simulink model "estimarParametros"  (R2021a)
settings: Solver=VariableStepAuto  StartTime=0.0  StopTime=10.0  RelTol=1e-3
values from neighbouring files (symbols this model uses):
  Bl0 = 0.0647    [modeloMatematico.m]    (also in motor copy.m = 0.147; motor.m = 0.05)
  Bm0 = 5.873e-9    (= 5.873e-09)    [modeloMatematico.m]    (also in motor copy.m = 5.862e-09; motor.m = 0.2)
  CL = double(subs(C_par))    [modeloMatematico.m]    (also in motor copy.m = [0 0 1/n0]; motor.m = [0 0 1/n0]; untitled.m = double(subs(C,{x1,x2,x3,u,M,g,R,L},{x10n,x20n,x30n,u0n,Mo,go)
  d0 = 0.065    [modeloMatematico.m]    (also in motor copy.m = 0.06587; motor.m = 0.1)
  g0 = 9.81    [modeloMatematico.m]    (also in motor copy.m; motor.m)
  Jl0 = 0.00000220756    (= 2.20756e-06)    [modeloMatematico.m]    (also in motor copy.m = 0.154364; motor.m = 0.02)
  Jm0 = 7.83568e-12    [modeloMatematico.m]    (also in motor copy.m = 7.83067e-12; motor.m = 0.01)
  Ki0 = 0.005119    [modeloMatematico.m]    (also in motor copy.m = 0.005012; motor.m = 2.3)
  Kv0 = 0.005119    [modeloMatematico.m]    (also in motor copy.m = 3.212e-11; motor.m = 1.5)
  L0 = 0.0013    [modeloMatematico.m]    (also in motor copy.m = 0.00051; motor.m = 0.04)
  m0 = 0.17244    [modeloMatematico.m]    (also in motor copy.m = 0.1045; motor.m = 0.1)
  n0 = 120    [modeloMatematico.m]    (also in motor copy.m; motor.m)
  R0 = 3.4    [modeloMatematico.m]    (also in motor copy.m = 3.9654; motor.m = 10)
  Vin0 = R0*x10    [modeloMatematico.m]    (also in motor copy.m; motor.m = R*x10)
  x10 = (m0*g0*d0*sin(x30))/Ki0    [modeloMatematico.m]    (also in motor copy.m = (m0*g0*d0*sin(x30/n0))/Ki0; motor.m = (m*g*d*sin(x30/n0))/Ki0)
  x20 = 0    [modeloMatematico.m]    (also in motor copy.m; motor.m; untitled.m)
  x30 = thetaL0    (= 0)    [modeloMatematico.m]    (also in motor copy.m; motor.m; untitled.m = sqrt(M*g*x10))
settings Model: OrderedModelArguments=off  Creator=hubertdelgado  LastModifiedBy=hubertdelgado

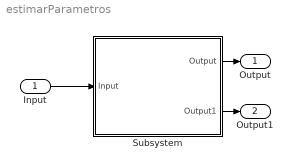
== system estimarParametros ==
  Input : Inport
  Subsystem : Subsystem
  Output : Outport
  Output1 : Outport  Port=2
  wires:
  Input/1 -> Subsystem/1(Input)
  Subsystem/1(Output) -> Output/1
  Subsystem/2(Output1) -> Output1/1

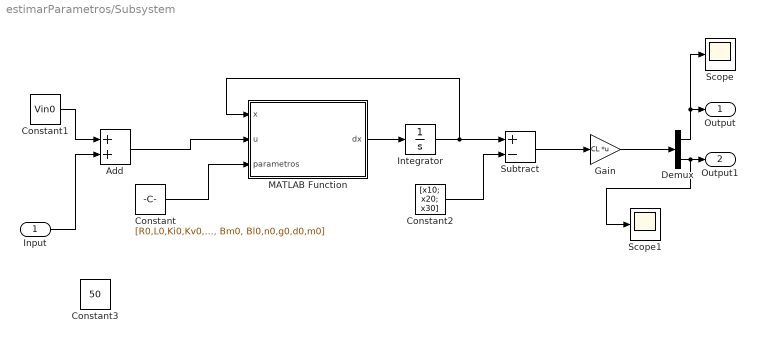
== system estimarParametros/Subsystem ==
  Input : Inport
  Add : Sum
  Constant : Constant  Value=[R0,L0,Ki0,Kv0,Jm0, Jl0, Bm0, Bl0,n0,g0,d0,m0]
  Constant1 : Constant  Value=Vin0
  Constant2 : Constant  Value=[x10; x20; x30]
  Constant3 : Constant  Value=50
  Demux : Demux  Outputs=2
  Gain : Gain  Gain=CL  Multiplication=Matrix(K*u)
  Integrator : Integrator  InitialCondition=[x10; x20; x30]
  MATLAB Function : MATLAB Function  TreatAsAtomicUnit=on
  Scope : Scope
  Scope1 : Scope
  Subtract : Sum  Inputs=+-
  Output : Outport
  Output1 : Outport  Port=2
  wires:
  Integrator/1 -> Subtract/1, MATLAB Function/1(x)
  Constant/1 -> MATLAB Function/3(parametros)
  Constant1/1 -> Add/1
  Constant2/1 -> Subtract/2
  MATLAB Function/1(dx) -> Integrator/1
  Add/1 -> MATLAB Function/2(u)
  Subtract/1 -> Gain/1
  Gain/1 -> Demux/1
  Demux/1 -> Scope/1, Output/1
  Demux/2 -> Scope1/1, Output1/1
  Input/1 -> Add/2

== matlab function estimarParametros/Subsystem/MATLAB Function ==
  data: x input; u input; dx output; parametros input
function dx = fcn(x,u,parametros)

x1 = x(1);
x2 = x(2);
x3 = x(3);
PWM = u;
Vin = 7*PWM/100;

R = parametros(1);
L = parametros(2);
Ki = parametros(3);
Kv = parametros(4);
Jm = parametros(5);
Jl = parametros(6);
Bm = parametros(7);
Bl = parametros(8);
n = parametros(9);
g = parametros(10);
d = parametros(11);
m = parametros(12);

Jt = Jm + (Jl/n^2);
f1 = (1/L)*(Vin - R*x1 - Kv*x2);
f2 = (1/Jt)*(Ki*x1 - (Bm + Bl/n^2)*x2 - (m*g*d*sin(x3/n))/n);
f3 = x2;
dx = [f1; f2; f3];
